simulink model "ASK_2"  (Simulink 9.0)
settings: Solver=VariableStepAuto  StartTime=0.0  StopTime=10  MaxStep=0.01  MinStep=0.001  RelTol=1e-3
libraries: dsparch4 x2, commchan3 x1, commsink2 x1
settings Model: Creator=ayadd  LastModifiedBy=ayadd
settings SolverCC: ShapePreserveControl=EnableAll  ZeroCrossAlgorithm=Adaptive
settings DataIOCC: SaveFormat=Dataset
settings OptimizationCC: LifeSpan=auto
settings DebuggingCC: UnderspecifiedInitializationDetection=Simplified  MergeDetectMultiDrivingBlocksExec=error  SFUnexpectedBacktrackingDiag=error  SFNoUnconditionalDefaultTransitionDiag=error  SFExecutionAtInitializationDiag=warning
settings HardwareCC: ProdBitPerPointer=64  ProdBitPerSizeT=64  ProdBitPerPtrDiffT=64  ProdLargestAtomicFloat=Float  ProdIntDivRoundTo=Zero  ProdEndianess=LittleEndian  ProdWordSize=64  ProdHWDeviceType=Intel->x86-64 (Windows64)
settings ModelReferenceCC: PropagateSignalLabelsOutOfModel=on
settings CodeAppCC: StateflowObjectComments=off
settings GRTTargetCC: TargetLangStandard=C99 (ISO)
settings ConfigComp: CovMetricSettings=dwe  CovHtmlReporting=off  CovSaveCumulativeToWorkspaceVar=off  CovSaveSingleToWorkspaceVar=off  CovExternalEMLEnable=on

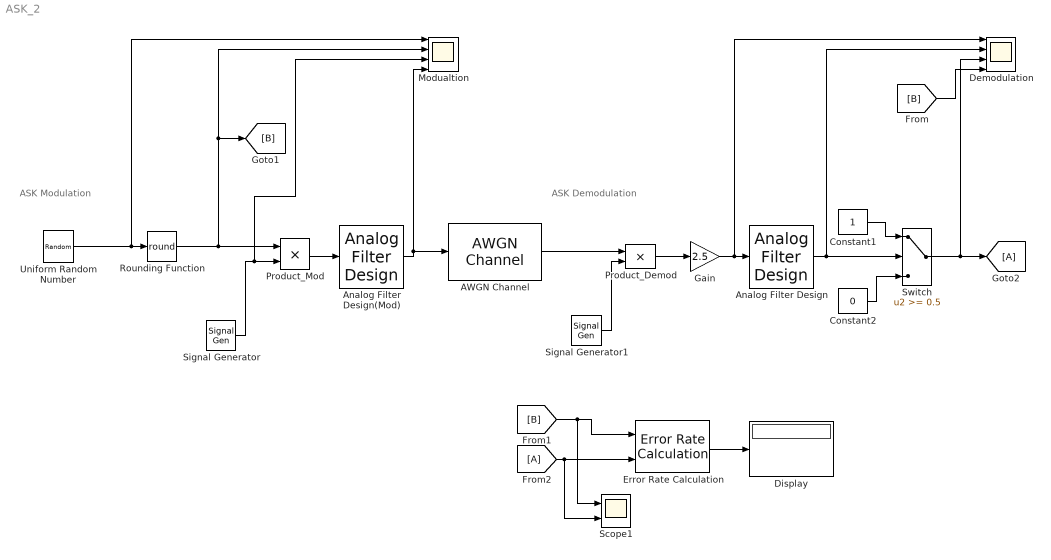
== system ASK_2 ==
  note: ASK Demodulation
  note: ASK Modulation
  AWGN Channel : commchan3/AWGN Channel  InputProcessing=Columns as channels (frame based)  seed=67  noiseMode="Signal to noise ratio  (SNR)"  EbNodB=10  EsNodB=10  SNRdB=30  bitsPerSym=1  Ps=1  Tsym=1  variance=1
  Analog Filter Design : dsparch4/Analog Filter Design  method=Butterworth  filttype=Lowpass  N=8  Wlo=30  Whi=80  Rp=2  Rs=40
  Analog Filter Design(Mod) : dsparch4/Analog Filter Design  method=Butterworth  filttype=Bandpass  N=8  Wlo=1/(2*pi)  Whi=800/(2*pi)  Rp=2  Rs=40
  Constant1 : Constant
  Constant2 : Constant  Value=0
  Demodulation : Scope  NumInputPorts=4
  Display : Display
  Error Rate Calculation : commsink2/Error Rate Calculation  N=0  st_delay=0  cp_mode=Entire frame  subframe=[]  PMode=Port  WsName=ErrorVec  RsMode2=off  stop=off  numErr=100  maxBits=1e6
  Gain : Gain  Gain=2.5
  Modualtion : Scope  NumInputPorts=4
  Product_Demod : Product  SaturateOnIntegerOverflow=on  InputSameDT=on  OutDataTypeStr=Inherit: Same as first input
  Product_Mod : Product
  Rounding Function : Rounding  Operator=round
  Scope1 : Scope  NumInputPorts=2
  Signal Generator : SignalGenerator  Frequency=4
  Signal Generator1 : SignalGenerator  Frequency=4
  Switch : Switch  Threshold=0.5  RndMeth=Round  SaturateOnIntegerOverflow=on  InputSameDT=on
  Uniform Random Number : UniformRandomNumber  Minimum=0  SampleTime=1
  wires:
  Uniform Random Number/1 -> Modualtion/1, Rounding Function/1
  Signal Generator/1 -> Product_Mod/2, Modualtion/3
  Signal Generator1/1 -> Product_Demod/2
  Product_Demod/1 -> Gain/1
  Analog Filter Design/1 -> Switch/2, Demodulation/2
  Gain/1 -> Demodulation/1, Analog Filter Design/1
  Rounding Function/1 -> Product_Mod/1, [B], Modualtion/2
  AWGN Channel/1 -> Product_Demod/1
  [B] -> Demodulation/4
  [B] -> Scope1/1, Error Rate Calculation/1
  [A] -> Scope1/2, Error Rate Calculation/2
  Error Rate Calculation/1 -> Display/1
  Switch/1 -> Demodulation/3, [A]
  Constant1/1 -> Switch/1
  Constant2/1 -> Switch/3
  Product_Mod/1 -> Analog Filter Design(Mod)/1
  Analog Filter Design(Mod)/1 -> Modualtion/4, AWGN Channel/1
